simulink model "HVModAL_Fahrzeugmodell"  (R2015b)
settings: Solver=ode1  StartTime=0  StopTime=drp.driving_cycle.tstop  FixedStep=sim_params.Ts  RelTol=1e-5
PreLoadFcn:
  | % Add paths
  | addpath data
  | addpath(genpath('library'))
StartFcn:
  | Simulation.StartTime = tic;
StopFcn:
  | Simulation.DurationTime = toc(Simulation.StartTime);
undefined symbols (not defined in the file or in its folder): Batteries, BMS, BMS_Bat_, C_Nenn_DCDC1, C_Nenn_DCDC2, d2d, DC, DCDC_Converter_efficiency, DcDc_Converters, Dcl, drp, drv, elm, gen, gin, Hdc, hdc, HV, hvb, Hvb, ice, ldc, lib_dcl, lib_hdc, lib_hvb, lib_veh, Link, lossestable, mask_LUT_OCV, mask_LUT_OCV_SOC, mask_LUT_OCV_Temperature, mask_LUT_R, mask_LUT_Rs, mask_LUT_Rs_SOC, mask_LUT_Rs_Temperature, sim_params, speedvec, torquevec, tri, veh, Veh, Vehicle_Chassis
libraries: simulink x29, lib_tri_modules x7, lib_hdc_module x5, lib_gearbox x4, lib_hvb_battery_pack x3, cstblocks x3, PowerLimitBlock x2, MultiCellLibrary x2, lib_aux x1, lib_drv x1, lib_gen x1, lib_elm x1
(part 7 of 7)

== system HVModAL_Fahrzeugmodell/Energy Manager (Emg)/Battery Control/Driving_Mode/Range_extender 2/dynamic/power_distribution_new/power_follow_control ==
  note: #new#:
      | P_load-P_Bat2_max>0: --> P_load>P_Bat2_max --> P2=P_Bat2_max; P1=P_load-P2; discharge
      |
      | P_load-P_Bat2_max<0: --> 1): 0<P_load<P_Bat2_max -->P2=P_load*3; P1=P_load-P2; charged or (0<P_load<P_Bat2_max -->P2=P_load; P1=0;)
      |
      | 2): P_load<0 --> P2=|P_load|&P2<=P_Bat2_max; P1=P_load+P2; charged
  note: #previous#:
      | P_load-P_Bat2_max>0: --> P_load>P_Bat2_max --> P2=P_Bat2_max; P1=P_load-P2; discharge
      |
      | P_load-P_Bat2_max<0: --> 1): 0<P_load<P_Bat2_max -->P2=P_Bat2_max; P1=P_load-P2; charged
      |
      | 2): P_load<0 --> P2=P_Bat2_max; P1=P_load+P2; charged
  P_load : Inport
  P_Bat2_discharge_max : Inport  Port=2
  Constant1 : Constant  Value=0
  Gain : Gain  Gain=-1
  Gain1 : Gain  Gain=5
  P_Bat2_new : Scope  NumInputPorts=2
  P_Bat2_old : Scope  NumInputPorts=2
  P_UB_Bat1#2 : Scope
  Saturation1 : Saturate  UpperLimit=0  LowerLimit=-inf
  Subtract1 : Sum  Inputs=+-
  Subtract2 : Sum  Inputs=+-
  Subtract3 : Sum  Inputs=+-
  Switch{1,3..5} (4 alike) : Switch
  Switch2 : Switch  Threshold=5
  P_Bat2 : Outport
  wires:
  Switch1/1 -> P_Bat2/1, P_Bat2_new/2
  P_Bat2_discharge_max/1 -> Subtract2/2, Switch5/1, P_UB_Bat1#2/1, Switch1/1, Subtract3/2, Switch2/1
  Constant1/1 -> Switch2/3
  Switch2/1 -> Subtract1/2, Switch3/1
  Subtract1/1 -> Switch3/2
  Switch3/1 -> Switch4/1, Switch4/2
  Saturation1/1 -> Gain/1
  Gain/1 -> Switch5/3, Subtract2/1
  Subtract2/1 -> Switch5/2
  Switch5/1 -> Switch4/3
  Subtract3/1 -> Switch1/2
  Gain1/1 -> Switch1/3, Subtract3/1
  Switch4/1 -> P_Bat2_old/2, Gain1/1
  P_load/1 -> Switch2/2, Saturation1/1, Switch3/3, Subtract1/1, P_Bat2_new/1, P_Bat2_old/1

== system HVModAL_Fahrzeugmodell/Energy Manager (Emg)/Battery Control/Driving_Mode/Range_extender 2/dynamic/power_distribution_new/prevent_bat1_overcharge&& temperature control ==
  note: p_bat2_now= p_bat2 + overcharge_power (negative)
  note: Compare whether P_Bat1 beyond the limit P_max_charge
      | P_Bat1 - P_Bat1_max_charge (negative)
      | = positive --> normal charge
      | = negative --> overcharge
  note: p_bat1_max_charge (negative)
  note: P_Bat1=P_load-P_bat2
  note: <0 overcharge
  "P_load " : Inport
  P_bat2 : Inport  Port=2
  T_Cell_avg : Inport  Port=3
  Constant1 : Constant  Value=0
  Constant3 : Constant  Value=hvb.Bat1.P_max_cha
  Gain : Gain  Gain=-1
  Relational Operator4 : RelationalOperator  OutDataTypeStr=boolean
  Saturation : Saturate  UpperLimit=hvb.Bat2.P_max_disch  LowerLimit=0
  Subtract1 : Sum  Inputs=+-
  Subtract2 : Sum  Inputs=+-
  Subtract3 : Sum
  Switch1 : Switch  Criteria=u2 > Threshold
  Switch3 : Switch  Criteria=u2 > Threshold
  T_threshold : Constant  Value=-20
  "p_pat2_new " : Outport
  wires:
  Constant3/1 -> Gain/1
  Subtract2/1 -> Switch3/2, Subtract3/2
  Gain/1 -> Subtract2/2
  "P_load "/1 -> Subtract1/1
  Subtract1/1 -> Subtract2/1
  Subtract3/1 -> Saturation/1
  Saturation/1 -> Switch3/3
  P_bat2/1 -> Subtract1/2, Switch3/1, Subtract3/1
  T_threshold/1 -> Relational Operator4/2
  Relational Operator4/1 -> Switch1/2
  T_Cell_avg/1 -> Relational Operator4/1
  Switch1/1 -> "p_pat2_new "/1
  Switch3/1 -> Switch1/1
  Constant1/1 -> Switch1/3

== system HVModAL_Fahrzeugmodell/Energy Manager (Emg)/Battery Control/Driving_Mode/Range_extender 2/dynamic/soc estimination /SOC & I_rex  ==
  note: soc<30 => soc=30
  note: soc>79 => soc=100
  note: soc > 79%             convert to 100% (small difference between the effects of step-in soc 100% and 80% )
      | 79% > soc > 30%  stay
      | 30% > soc              convert to 30% (step-in soc lower than 30%, I_rex will be too high, Bat2 will be consumed too fast )
  note: To determine the current in each cell (I_rex) and the step-in soc
      | by different bat1 capacity and driving range
  E_bat1 : Inport
  speed : Inport  Port=2
  specific energy consumption : Inport  Port=3
  "cell " : Inport  Port=4
  driving range : Inport  Port=5
  Chart3 : Stateflow chart  TreatAsAtomicUnit=on
      settings: PermitHierarchicalResolution=ParametersOnly
  Constant5 : Constant  Value=100
  Constant8 : Constant  Value=30
  Display : Display
  Display1 : Display
  Saturation : Saturate  UpperLimit=hvb.Bat2.cell.I_max_disch  LowerLimit=0
  Scope{1,4,6..8,13} (6 alike) : Scope
  Switch2 : Switch  Criteria=u2 > Threshold  Threshold=79
  Switch4 : Switch  Criteria=u2 > Threshold  Threshold=30
  soc : Outport
  I_rex : Outport  Port=2
  wires:
  Constant5/1 -> Switch2/1
  Switch2/1 -> Switch4/1, Switch4/2
  Constant8/1 -> Switch4/3
  Switch4/1 -> soc/1
  speed/1 -> Chart3/2(speed)
  specific energy consumption/1 -> Chart3/3(E)
  Chart3/2(I_rex) -> Saturation/1
  Chart3/1(soc) -> Scope4/1, Switch2/3, Switch2/2
  Chart3/3(range) -> Scope6/1
  Chart3/4(range_2) -> Scope7/1
  Chart3/5(range_1) -> Scope8/1
  "cell "/1 -> Display1/1, Chart3/4(cell)
  E_bat1/1 -> Scope1/1, Chart3/1(E_bat1)
  Saturation/1 -> Scope13/1, I_rex/1
  driving range/1 -> Display/1, Chart3/5(driving_range)

== system HVModAL_Fahrzeugmodell/Energy Manager (Emg)/Battery Control/Driving_Mode/Range_extender 2/start_from_30% 1/power estimination /mapping1 ==
  P_max_ch_W_Bat1 : Inport
  P_max_Disch_W_Bat1 : Inport  Port=2
  Gain : Gain  Gain=-1
  P_LB_Bat1 : Outport
  P_UB_Bat1 : Outport  Port=2
  wires:
  Gain/1 -> P_LB_Bat1/1
  P_max_ch_W_Bat1/1 -> Gain/1
  P_max_Disch_W_Bat1/1 -> P_UB_Bat1/1

== system HVModAL_Fahrzeugmodell/Energy Manager (Emg)/Battery Control/Driving_Mode/Range_extender 2/start_from_30% 1/power_distribution_new/prevent_bat1_overcharge&& temperature control ==
  note: p_bat2_now= p_bat2_previous + overcharge_power (negative)
  note: p_bat1 - p_bat1_max_charge (negative)
      | = positive --> normal charge
      | = negative --> overcharge
  note: p_bat1_max_charge (negative)
  note: P_bat1=p_load-p_bat2
  note: <0 overcharge
  "p_load " : Inport
  p_bat2_previous : Inport  Port=2
  T_Cell_avg : Inport  Port=3
  Constant1 : Constant  Value=0
  Constant3 : Constant  Value=hvb.Bat1.P_max_cha
  Gain : Gain  Gain=-1
  Relational Operator4 : RelationalOperator  OutDataTypeStr=boolean
  Saturation : Saturate  UpperLimit=hvb.Bat2.P_max_disch  LowerLimit=0
  Scope : Scope
  Subtract1 : Sum  Inputs=+-
  Subtract2 : Sum  Inputs=+-
  Subtract3 : Sum
  Switch1 : Switch  Criteria=u2 > Threshold
  Switch3 : Switch  Criteria=u2 > Threshold
  T_threshold : Constant  Value=-20
  "p_pat2_now " : Outport
  wires:
  Constant3/1 -> Scope/1, Gain/1
  Subtract2/1 -> Switch3/2, Subtract3/2
  Gain/1 -> Subtract2/2
  "p_load "/1 -> Subtract1/1
  Subtract1/1 -> Subtract2/1
  Subtract3/1 -> Saturation/1
  Saturation/1 -> Switch3/3
  p_bat2_previous/1 -> Subtract1/2, Switch3/1, Subtract3/1
  Constant1/1 -> Switch1/3
  Relational Operator4/1 -> Switch1/2
  T_Cell_avg/1 -> Relational Operator4/1
  Switch1/1 -> "p_pat2_now "/1
  Switch3/1 -> Switch1/1
  T_threshold/1 -> Relational Operator4/2

== system HVModAL_Fahrzeugmodell/Energy Manager (Emg)/Battery Control/Driving_Mode/Range_extender 2/start_from_30% 1/soc estimination /Subsystem ==
  note: actual distance the rest capacity of bat1 can do
  note: rest distance
  soc_perc_bat1 : Inport
  E_bat1 : Inport  Port=2
  driving_range : Inport  Port=3
  V : Inport  Port=4
  % : Constant  Value=100
  5% soc rest : Constant  Value=5
  Add : Sum  Inputs=+-
  Add1 : Sum  Inputs=+-
  Constant3 : Constant  Value=1000
  Divide : Product  Inputs=*/
  Divide2 : Product  Inputs=**//
  Integrator : Integrator
  Relational Operator1 : RelationalOperator  Operator=>  OutDataTypeStr=boolean
  Scope : Scope
  energy consumption per km : Constant  Value=160
  only_bat1_capability : Outport
  wires:
  Divide/1 -> Add1/2, Scope/1
  soc_perc_bat1/1 -> Add/1
  Divide2/1 -> Relational Operator1/1
  Add1/1 -> Relational Operator1/2
  energy consumption per km/1 -> Divide2/4
  Add/1 -> Divide2/1
  %/1 -> Divide2/3
  5% soc rest/1 -> Add/2
  V/1 -> Integrator/1
  Relational Operator1/1 -> only_bat1_capability/1
  Constant3/1 -> Divide/2
  Integrator/1 -> Divide/1
  driving_range/1 -> Add1/1
  E_bat1/1 -> Divide2/2

== system HVModAL_Fahrzeugmodell/Energy Manager (Emg)/Battery Control/Driving_Mode/Range_extender 2/start_from_begining /power estimination /mapping1 ==
  P_max_ch_W_Bat1 : Inport
  P_max_Disch_W_Bat1 : Inport  Port=2
  Gain : Gain  Gain=-1
  P_LB_Bat1 : Outport
  P_UB_Bat1 : Outport  Port=2
  wires:
  Gain/1 -> P_LB_Bat1/1
  P_max_ch_W_Bat1/1 -> Gain/1
  P_max_Disch_W_Bat1/1 -> P_UB_Bat1/1

== system HVModAL_Fahrzeugmodell/Energy Manager (Emg)/Battery Control/Driving_Mode/Range_extender 2/start_from_begining /power_distribution_new/power_follow_control ==
  note: #new#:
      | P_load-P_Bat2_max>0: --> P_load>P_Bat2_max --> P2=P_Bat2_max; P1=P_load-P2; discharge
      |
      | P_load-P_Bat2_max<0: --> 1): 0<P_load<P_Bat2_max -->P2=P_load*3; P1=P_load-P2; charged or (0<P_load<P_Bat2_max -->P2=P_load; P1=0;)
      |
      | 2): P_load<0 --> P2=|P_load|&P2<=P_Bat2_max; P1=P_load+P2; charged
  note: #previous#:
      | P_load-P_Bat2_max>0: --> P_load>P_Bat2_max --> P2=P_Bat2_max; P1=P_load-P2; discharge
      |
      | P_load-P_Bat2_max<0: --> 1): 0<P_load<P_Bat2_max -->P2=P_Bat2_max; P1=P_load-P2; charged
      |
      | 2): P_load<0 --> P2=P_Bat2_max; P1=P_load+P2; charged
  P_load : Inport
  P_Bat2_discharge_max : Inport  Port=2
  Constant1 : Constant  Value=0
  Gain : Gain  Gain=-1
  Gain1 : Gain
  P_Bat2_new : Scope  NumInputPorts=2
  P_Bat2_old : Scope  NumInputPorts=2
  P_UB_Bat1#2 : Scope
  Saturation1 : Saturate  UpperLimit=0  LowerLimit=-inf
  Subtract1 : Sum  Inputs=+-
  Subtract2 : Sum  Inputs=+-
  Subtract3 : Sum  Inputs=+-
  Switch{1,3..5} (4 alike) : Switch
  Switch2 : Switch  Threshold=5
  P_Bat2 : Outport
  wires:
  Switch1/1 -> P_Bat2/1, P_Bat2_new/2
  P_Bat2_discharge_max/1 -> Subtract2/2, Switch5/1, P_UB_Bat1#2/1, Switch1/1, Subtract3/2, Switch2/1
  Constant1/1 -> Switch2/3
  Switch2/1 -> Subtract1/2, Switch3/1
  Subtract1/1 -> Switch3/2
  Switch3/1 -> Switch4/1, Switch4/2
  Saturation1/1 -> Gain/1
  Gain/1 -> Switch5/3, Subtract2/1
  Subtract2/1 -> Switch5/2
  Switch5/1 -> Switch4/3
  Subtract3/1 -> Switch1/2
  Gain1/1 -> Switch1/3, Subtract3/1
  Switch4/1 -> P_Bat2_old/2, Gain1/1
  P_load/1 -> Switch2/2, Saturation1/1, Switch3/3, Subtract1/1, P_Bat2_new/1, P_Bat2_old/1

== system HVModAL_Fahrzeugmodell/Energy Manager (Emg)/Battery Control/Driving_Mode/Range_extender 2/start_from_begining /power_distribution_new/prevent_bat1_overcharge&& temperature control ==
  note: p_bat2_new= p_bat2_old + overcharge_power (negative)
  note: p_bat1 - p_bat1_max_charge (negative)
      | = positive --> normal charge
      | = negative --> overcharge
  note: p_bat1_max_charge (negative)
  note: P_bat1=p_load-p_bat2
  note: <0 overcharge
  "p_load " : Inport
  p_bat2_old : Inport  Port=2
  T_Cell_avg : Inport  Port=3
  Constant1 : Constant  Value=0
  Constant3 : Constant  Value=hvb.Bat1.P_max_cha
  Gain : Gain  Gain=-1
  Relational Operator4 : RelationalOperator  OutDataTypeStr=boolean
  Saturation : Saturate  UpperLimit=hvb.Bat2.P_max_disch  LowerLimit=0
  Subtract1 : Sum  Inputs=+-
  Subtract2 : Sum  Inputs=+-
  Subtract3 : Sum
  Switch1 : Switch  Criteria=u2 > Threshold
  Switch3 : Switch  Criteria=u2 > Threshold
  T_threshold : Constant  Value=-20
  "p_pat2_new " : Outport
  wires:
  Constant3/1 -> Gain/1
  Subtract2/1 -> Switch3/2, Subtract3/2
  Gain/1 -> Subtract2/2
  "p_load "/1 -> Subtract1/1
  Subtract1/1 -> Subtract2/1
  Subtract3/1 -> Saturation/1
  Saturation/1 -> Switch3/3
  p_bat2_old/1 -> Subtract1/2, Switch3/1, Subtract3/1
  Constant1/1 -> Relational Operator4/2
  Relational Operator4/1 -> Switch1/2
  T_Cell_avg/1 -> Relational Operator4/1
  Switch1/1 -> "p_pat2_new "/1
  Switch3/1 -> Switch1/1
  T_threshold/1 -> Switch1/3

== system HVModAL_Fahrzeugmodell/Energy Manager (Emg)/Battery Control/Driving_Mode/Strategy_Maximiziation_Driving_Range1/Minloss Strategy/Sufficient Energy left/SOC Management ==
  Pload : Inport
  R1 : Inport  Port=2
  R2 : Inport  Port=3
  V1 : Inport  Port=4
  V2 : Inport  Port=5
  P_max_disch_bat1 : Inport  Port=6
  P_max_char_bat2 : Inport  Port=7
  P_max_disch_bat2 : Inport  Port=8
  P_max_char_bat1 : Inport  Port=9
  Enable : EnablePort
  Acceleration : Subsystem
  Compare To Zero : simulink/Logic and Bit Operations/Compare To Zero  relop=>  OutDataTypeStr=boolean
  L : Logic  Operator=NOT  AllPortsSameDT=off  OutDataTypeStr=boolean
  Merge : Merge
  Merge1 : Merge
  Recuperation : Subsystem
  vector_PowerDistribution : Outport
  P_exchange_Master_Slave : Outport  Port=2
  wires:
  Recuperation/2(P_exchange_Master_Slave) -> Merge1/2
  Acceleration/2(P_exchange_Master_Slave) -> Merge1/1
  Merge1/1 -> P_exchange_Master_Slave/1
  Merge/1 -> vector_PowerDistribution/1
  Pload/1 -> Compare To Zero/1, Recuperation/5(Pload)
  P_max_char_bat2/1 -> Acceleration/6(P_max_char_bat2), Recuperation/2(P_max_char_bat2)
  P_max_char_bat1/1 -> Recuperation/4(P_max_char_bat1)
  P_max_disch_bat2/1 -> Recuperation/3(P_max_disch_bat2)
  Recuperation/1(vector_PowerDistribution) -> Merge/2
  L/1 -> Recuperation/Enable
  Compare To Zero/1 -> Acceleration/Enable, L/1
  Acceleration/1(vector_PowerDistribution) -> Merge/1
  P_max_disch_bat1/1 -> Acceleration/5(P_max_disch_bat1), Recuperation/1(P_max_disch_bat1)
  V2/1 -> Acceleration/4(V2)
  V1/1 -> Acceleration/3(V1)
  R2/1 -> Acceleration/2(R2)
  R1/1 -> Acceleration/1(R1)

== system HVModAL_Fahrzeugmodell/Energy Manager (Emg)/Battery Control/Driving_Mode/Strategy_Maximiziation_Driving_Range1/Minloss Strategy/Sufficient Energy left/SOC Management/Acceleration ==
  R1 : Inport
  R2 : Inport  Port=2
  V1 : Inport  Port=3
  V2 : Inport  Port=4
  P_max_disch_bat1 : Inport  Port=5
  P_max_char_bat2 : Inport  Port=6
  Enable : EnablePort
  Constant : Constant  Value=0
  Constant1 : Constant
  Constant2 : Constant  Value=0
  Gain : Gain  Gain=100
  Mux1 : Mux  Inputs=3
  N : Constant  Value=50
  Optimal charge power : Subsystem  TreatAsAtomicUnit=on
  vector_PowerDistribution : Outport
  P_exchange_Master_Slave : Outport  Port=2
  wires:
  Gain/1 -> vector_PowerDistribution/1
  Constant1/1 -> Mux1/1
  N/1 -> Optimal charge power/7(N)
  V2/1 -> Optimal charge power/4(V2)
  P_max_disch_bat1/1 -> Optimal charge power/5(P_max_disch_bat1)
  Mux1/1 -> Gain/1
  Constant2/1 -> Mux1/2
  R1/1 -> Optimal charge power/1("R1 ")
  Optimal charge power/1(P_trans) -> P_exchange_Master_Slave/1  "P_transferred"
  R2/1 -> Optimal charge power/2("R2 ")
  Constant/1 -> Mux1/3  "powershare_bat3"
  P_max_char_bat2/1 -> Optimal charge power/6(P_max_char_bat2)
  V1/1 -> Optimal charge power/3(V1)

== system HVModAL_Fahrzeugmodell/Energy Manager (Emg)/Battery Control/Driving_Mode/Strategy_Maximiziation_Driving_Range1/Minloss Strategy/Sufficient Energy left/SOC Management/Recuperation ==
  P_max_disch_bat1 : Inport
  P_max_char_bat2 : Inport  Port=2
  P_max_disch_bat2 : Inport  Port=3
  P_max_char_bat1 : Inport  Port=4
  Pload : Inport  Port=5
  Enable : EnablePort
  Constant : Constant  Value=0
  Constant1 : Constant  Value=0
  Constant2 : Constant
  Constant3 : Constant  Value=0
  Gain : Gain  Gain=100
  Mux1 : Mux  Inputs=3
  Power Limit1 : PowerLimitBlock/Power Limit
  Saturation : Saturate  UpperLimit=-0.001  LowerLimit=-inf
  vector_PowerDistribution : Outport
  P_exchange_Master_Slave : Outport  Port=2
  wires:
  Constant3/1 -> P_exchange_Master_Slave/1
  Gain/1 -> vector_PowerDistribution/1
  Saturation/1 -> Power Limit1/7
  Constant2/1 -> Power Limit1/6
  Constant1/1 -> Power Limit1/5
  Pload/1 -> Saturation/1
  Constant/1 -> Mux1/3
  Power Limit1/2 -> Mux1/2
  Power Limit1/1 -> Mux1/1
  P_max_char_bat1/1 -> Power Limit1/2
  P_max_disch_bat2/1 -> Power Limit1/3
  P_max_char_bat2/1 -> Power Limit1/4
  P_max_disch_bat1/1 -> Power Limit1/1
  Mux1/1 -> Gain/1

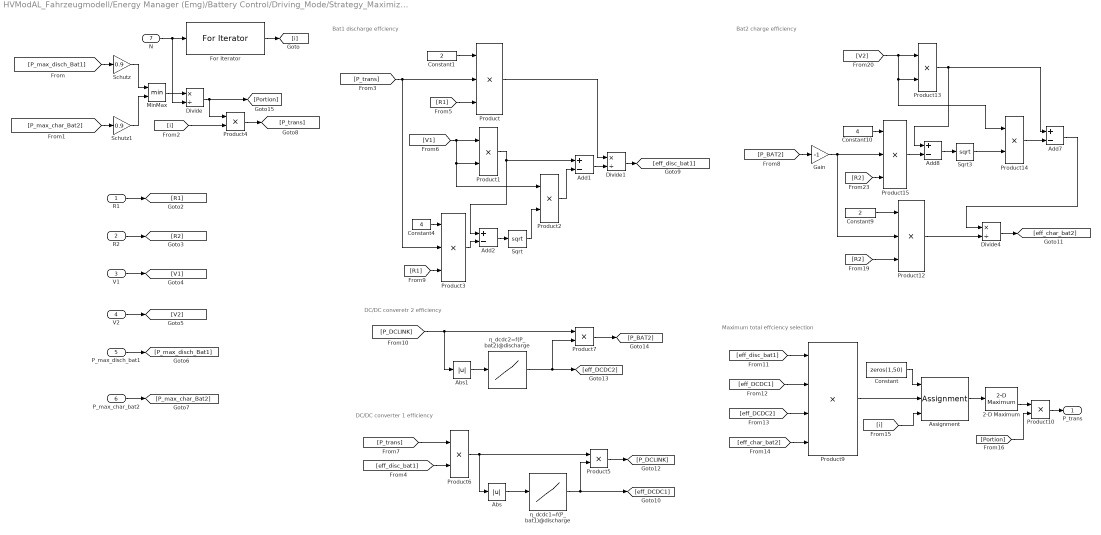
== system HVModAL_Fahrzeugmodell/Energy Manager (Emg)/Battery Control/Driving_Mode/Strategy_Maximiziation_Driving_Range1/Minloss Strategy/Sufficient Energy left/SOC Management/Acceleration/Optimal charge power ==
  note: Bat1 discharge effciency
  note: Bat2 charge efficiency
  note: Maximum total effciency selection
  note: DC/DC converter 1 efficiency
  note: DC/DC converetr 2 efficiency
  "R1 " : Inport
  "R2 " : Inport  Port=2
  V1 : Inport  Port=3
  V2 : Inport  Port=4
  P_max_disch_bat1 : Inport  Port=5
  P_max_char_bat2 : Inport  Port=6
  N : Inport  Port=7
  2-D Maximum : visionstatistics/2-D Maximum  fcn=Value and Index  reset=None  indexBase=One  operateOver=Entire input  Dimension=1  colComp=on  operation=maximum  roiEnable=off  roiType=Rectangles  roiPortion=Entire ROI  roiOutput=Individual statistics for each ROI  roiFlag=off  accumDataTypeStr=Inherit: Same as product output  accumLastDataTypeStr=Inherit: Same as product output  roundingMode=Floor  overflowMode=off
  Abs : Abs
  Abs1 : Abs
  Add{1..2,7..8} (4 alike) : Sum  Inputs=+-
  Assignment : Assignment  DiagnosticForDimensions=Warning  IndexOptions=Index vector (port)  Indices=1  OutputSizes=1
  Constant : Constant  Value=zeros(1,50)
  Constant1 : Constant  Value=2
  Constant10 : Constant  Value=4
  Constant4 : Constant  Value=4
  Constant9 : Constant  Value=2
  Divide : Product  Inputs=*/
  Divide1 : Product  Inputs=*/
  Divide4 : Product  Inputs=*/
  For Iterator : ForIterator  IterationSource=external
  Gain : Gain  Gain=-1
  MinMax : MinMax  Inputs=2
  Product{,3,12,15} (4 alike) : Product  Inputs=3
  Product{1..2,4..7,10,13..14} (9 alike) : Product
  Product9 : Product  Inputs=4
  Schutz : Gain  Gain=0.9
  Schutz1 : Gain  Gain=0.9
  Sqrt : Sqrt  SaturateOnIntegerOverflow=on
  Sqrt3 : Sqrt  SaturateOnIntegerOverflow=on
  η_dcdc1=f(P_bat1)@discharge : Lookup_n-D  NumberOfTableDimensions=1  BreakpointsForDimension1=DCDC_Converter_efficiency(1,1:8)*C_Nenn_DCDC1  Table=DCDC_Converter_efficiency(2,1:8)  ExtrapMethod=Clip  UseLastTableValue=on  InternalRulePriority=Speed  RndMeth=Simplest  InputSameDT=on
  η_dcdc2=f(P_bat2)@discharge : Lookup_n-D  NumberOfTableDimensions=1  BreakpointsForDimension1=DCDC_Converter_efficiency(1,1:8)*C_Nenn_DCDC2  Table=DCDC_Converter_efficiency(2,1:8)  ExtrapMethod=Clip  UseLastTableValue=on  InternalRulePriority=Speed  RndMeth=Simplest  InputSameDT=on
  P_trans : Outport
  wires:
  Add1/1 -> Divide1/2
  Add2/1 -> Sqrt/1
  Divide4/1 -> [eff_char_bat2]
  Gain/1 -> Product15/2, Product12/2
  Product6/1 -> Product5/1, Abs/1
  Abs/1 -> η_dcdc1=f(P_bat1)@discharge/1
  Product4/1 -> [P_trans]
  [eff_char_bat2] -> Product9/4
  [eff_DCDC2] -> Product9/3
  [eff_DCDC1] -> Product9/2
  Product10/1 -> P_trans/1
  [Portion] -> Product10/2
  2-D Maximum/2 -> Product10/1
  Assignment/1 -> 2-D Maximum/1
  Constant/1 -> Assignment/1
  [i] -> Assignment/3
  Product9/1 -> Assignment/2
  [eff_disc_bat1] -> Product9/1
  Product7/1 -> [P_BAT2]
  [P_DCLINK] -> Product7/1, Abs1/1
  η_dcdc2=f(P_bat2)@discharge/1 -> Product7/2, [eff_DCDC2]
  Abs1/1 -> η_dcdc2=f(P_bat2)@discharge/1
  [P_trans] -> Product6/1
  [eff_disc_bat1] -> Product6/2
  Product5/1 -> [P_DCLINK]
  η_dcdc1=f(P_bat1)@discharge/1 -> Product5/2, [eff_DCDC1]
  [i] -> Product4/2
  Divide/1 -> Product4/1, [Portion]
  MinMax/1 -> Divide/1
  Schutz1/1 -> MinMax/2
  Schutz/1 -> MinMax/1
  [P_max_char_Bat2] -> Schutz1/1
  [P_max_disch_Bat1] -> Schutz/1
  P_max_char_bat2/1 -> [P_max_char_Bat2]
  P_max_disch_bat1/1 -> [P_max_disch_Bat1]
  Divide1/1 -> [eff_disc_bat1]
  Constant1/1 -> Product/1
  Product12/1 -> Divide4/2
  Add7/1 -> Divide4/1
  [R2] -> Product15/3
  Constant10/1 -> Product15/1
  Product15/1 -> Add8/2
  Add8/1 -> Sqrt3/1
  Sqrt3/1 -> Product14/2
  Product14/1 -> Add7/2
  Product13/1 -> Add7/1, Add8/1
  [V2] -> Product13/2, Product14/1, Product13/1
  [R2] -> Product12/3
  [P_BAT2] -> Gain/1
  Constant9/1 -> Product12/1
  [R1] -> Product3/3
  Constant4/1 -> Product3/1
  [P_trans] -> Product/2, Product3/2
  Product3/1 -> Add2/2
  Sqrt/1 -> Product2/2
  Product2/1 -> Add1/2
  Product1/1 -> Add2/1, Add1/1
  [V1] -> Product1/1, Product1/2, Product2/1
  [R1] -> Product/3
  Product/1 -> Divide1/1
  V2/1 -> [V2]
  V1/1 -> [V1]
  "R2 "/1 -> [R2]
  "R1 "/1 -> [R1]
  For Iterator/1 -> [i]
  N/1 -> Divide/2, For Iterator/1

== stateflow chart HVModAL_Fahrzeugmodell/Energy Manager (Emg)/Battery Control/Driving_Mode/Range_extender 1/Chart ==
  state start
    during:Use_Range_extender=0;
  state Not_use_Range_Extender
    during: Use_Range_extender=0;
  state Check_SOC_of_Battery_01
  state Check_SOC_of_Battery_02
  state Use_Range_Extender
    during: Use_Range_extender=1;
  (default) -> start
  start -> Check_SOC_of_Battery_01
  Check_SOC_of_Battery_01 -> Not_use_Range_Extender [order 2] : [SOC_perc_01>SOC_limit]
      | {Use_Range_extender=0;}
  Not_use_Range_Extender -> Check_SOC_of_Battery_02 : [SOC_perc_01<=SOC_limit]
  Use_Range_Extender -> Not_use_Range_Extender : [SOC_perc_01>(SOC_limit+1)]
      | {Use_Range_extender=0;}
  Check_SOC_of_Battery_02 -> Not_use_Range_Extender [order 2] : [SOC_perc_02==0]
      | {Use_Range_extender=0;}
  Check_SOC_of_Battery_01 -> Check_SOC_of_Battery_02 [order 1] : [SOC_perc_01<=SOC_limit]
  Check_SOC_of_Battery_02 -> Use_Range_Extender [order 1] : [SOC_perc_02>0]
      | {Use_Range_extender=1;}
  data: SOC_perc_01 input; Use_Range_extender output; SOC_perc_02 input; SOC_limit input
  events: event local FUNCTION_CALL_EVENT

== stateflow chart HVModAL_Fahrzeugmodell/Energy Manager (Emg)/Battery Control/Driving_Mode/Range_extender 1/power_distribution_old/Chart ==
  state start
    during:P_Bat1=p_Bat1_o;
  state P_LB_Bat1
  state P_UB_Bat1
  (default) -> start
  P_UB_Bat1 -> start [order 1] : [p_Bat1_o<P_UB_Bat1&&...
      | p_Bat1_o>P_LB_Bat1]
      | {P_Bat1=p_Bat1_o;}
  start -> P_UB_Bat1 [order 1] : [p_Bat1_o>P_UB_Bat1]
      | {P_Bat1=P_UB_Bat1;}
  start -> P_LB_Bat1 [order 2] : [p_Bat1_o<P_LB_Bat1]
      | {P_Bat1=P_LB_Bat1;}
  P_LB_Bat1 -> start [order 1] : [p_Bat1_o>P_LB_Bat1&&...
      | p_Bat1_o<P_UB_Bat1]
      | {P_Bat1=p_Bat1_o;}
  P_LB_Bat1 -> P_UB_Bat1 [order 2] : [p_Bat1_o>P_UB_Bat1]
      | {P_Bat1=P_UB_Bat1;}
  P_UB_Bat1 -> P_LB_Bat1 [order 2] : [p_Bat1_o<P_LB_Bat1]
      | {P_Bat1=P_LB_Bat1;}
  data: p_Bat1_o input; P_Bat1 output; P_UB_Bat1 input; P_LB_Bat1 input
  events: event local FUNCTION_CALL_EVENT

== stateflow chart HVModAL_Fahrzeugmodell/Energy Manager (Emg)/Battery Control/Driving_Mode/Range_extender 2/start_from_begining /power_distribution_new/Chart ==
  state start
    during:P_Bat1=p_Bat1_o;
  state P_LB_Bat1
  state P_UB_Bat1
  (default) -> start
  P_UB_Bat1 -> start [order 1] : [p_Bat1_o<P_UB_Bat1&&...
      | p_Bat1_o>P_LB_Bat1]
      | {P_Bat1=p_Bat1_o;}
  start -> P_UB_Bat1 [order 1] : [p_Bat1_o>P_UB_Bat1]
      | {P_Bat1=P_UB_Bat1;}
  start -> P_LB_Bat1 [order 2] : [p_Bat1_o<P_LB_Bat1]
      | {P_Bat1=P_LB_Bat1;}
  P_LB_Bat1 -> start [order 1] : [p_Bat1_o>P_LB_Bat1&&...
      | p_Bat1_o<P_UB_Bat1]
      | {P_Bat1=p_Bat1_o;}
  P_LB_Bat1 -> P_UB_Bat1 [order 2] : [p_Bat1_o>P_UB_Bat1]
      | {P_Bat1=P_UB_Bat1;}
  P_UB_Bat1 -> P_LB_Bat1 [order 2] : [p_Bat1_o<P_LB_Bat1]
      | {P_Bat1=P_LB_Bat1;}
  data: p_Bat1_o input; P_Bat1 output; P_UB_Bat1 input; P_LB_Bat1 input
  events: event local FUNCTION_CALL_EVENT

== stateflow chart HVModAL_Fahrzeugmodell/Energy Manager (Emg)/Battery Control/Driving_Mode/Range_extender 2/start_from_30% 1/power_distribution_new/Chart ==
  state start
    during:P_Bat1=p_Bat1_o;
  state P_LB_Bat1
  state P_UB_Bat1
  (default) -> start
  P_UB_Bat1 -> start [order 1] : [p_Bat1_o<P_UB_Bat1&&...
      | p_Bat1_o>P_LB_Bat1]
      | {P_Bat1=p_Bat1_o;}
  start -> P_UB_Bat1 [order 1] : [p_Bat1_o>P_UB_Bat1]
      | {P_Bat1=P_UB_Bat1;}
  start -> P_LB_Bat1 [order 2] : [p_Bat1_o<P_LB_Bat1]
      | {P_Bat1=P_LB_Bat1;}
  P_LB_Bat1 -> start [order 1] : [p_Bat1_o>P_LB_Bat1&&...
      | p_Bat1_o<P_UB_Bat1]
      | {P_Bat1=p_Bat1_o;}
  P_LB_Bat1 -> P_UB_Bat1 [order 2] : [p_Bat1_o>P_UB_Bat1]
      | {P_Bat1=P_UB_Bat1;}
  P_UB_Bat1 -> P_LB_Bat1 [order 2] : [p_Bat1_o<P_LB_Bat1]
      | {P_Bat1=P_LB_Bat1;}
  data: p_Bat1_o input; P_Bat1 output; P_UB_Bat1 input; P_LB_Bat1 input
  events: event local FUNCTION_CALL_EVENT

== stateflow chart HVModAL_Fahrzeugmodell/Energy Manager (Emg)/Battery Control/Driving_Mode/Range_extender 2/dynamic/soc estimination /Chart3 ==
  (default) -> (junction 52) : % while
  (junction 52) -> (junction 54) : {i=10;...
      | range=0;}
  (junction 54) -> (junction 53) [order 1] : [range<driving_range&&i<101]
  (junction 53) -> (junction 55) : {soc=i;...
      |  rest=soc*E_bat1/100;...
      |  range_1=rest/E;...
      | range_bat1=E_bat1/E;...
      |  t=range_1/speed;...
      |  I_rex=3.1/t;...
      |  e_rex=1/(0.216+0.0479*I_rex)*cell;...
      |  range_2=e_rex/E;...
      |  range=range_bat1+range_2;...
      |  i=i+10;  }
  (junction 55) -> (junction 54)
  (junction 54) -> (junction 56) [order 2]
  data: E_bat1 input; speed input; E input; cell input; t local; e_rex local; E_rex local; rest local; soc output; I_rex output; range output; i local; range_2 output; range_1 output; range_bat1 local; driving_range input

== stateflow chart HVModAL_Fahrzeugmodell/Energy Manager (Emg)/Battery Control/Driving_Mode/Range_extender 2/dynamic/power_distribution_new/Chart ==
  state start
    during:P_Bat1=p_Bat1_o;
  state P_LB_Bat1
  state P_UB_Bat1
  (default) -> start
  P_UB_Bat1 -> start [order 1] : [p_Bat1_o<P_UB_Bat1&&...
      | p_Bat1_o>P_LB_Bat1]
      | {P_Bat1=p_Bat1_o;}
  start -> P_UB_Bat1 [order 1] : [p_Bat1_o>P_UB_Bat1]
      | {P_Bat1=P_UB_Bat1;}
  start -> P_LB_Bat1 [order 2] : [p_Bat1_o<P_LB_Bat1]
      | {P_Bat1=P_LB_Bat1;}
  P_LB_Bat1 -> start [order 1] : [p_Bat1_o>P_LB_Bat1&&...
      | p_Bat1_o<P_UB_Bat1]
      | {P_Bat1=p_Bat1_o;}
  P_LB_Bat1 -> P_UB_Bat1 [order 2] : [p_Bat1_o>P_UB_Bat1]
      | {P_Bat1=P_UB_Bat1;}
  P_UB_Bat1 -> P_LB_Bat1 [order 2] : [p_Bat1_o<P_LB_Bat1]
      | {P_Bat1=P_LB_Bat1;}
  data: p_Bat1_o input; P_Bat1 output; P_UB_Bat1 input; P_LB_Bat1 input
  events: event local FUNCTION_CALL_EVENT

== stateflow chart HVModAL_Fahrzeugmodell/Energy Manager (Emg)/Battery Control/Driving_Mode/Range_extender 1/power_distribution_new/Chart ==
  state start
    during:P_Bat1=p_Bat1_o;
  state P_LB_Bat1
  state P_UB_Bat1
  (default) -> start
  P_UB_Bat1 -> start [order 1] : [p_Bat1_o<P_UB_Bat1&&...
      | p_Bat1_o>P_LB_Bat1]
      | {P_Bat1=p_Bat1_o;}
  start -> P_UB_Bat1 [order 1] : [p_Bat1_o>P_UB_Bat1]
      | {P_Bat1=P_UB_Bat1;}
  start -> P_LB_Bat1 [order 2] : [p_Bat1_o<P_LB_Bat1]
      | {P_Bat1=P_LB_Bat1;}
  P_LB_Bat1 -> start [order 1] : [p_Bat1_o>P_LB_Bat1&&...
      | p_Bat1_o<P_UB_Bat1]
      | {P_Bat1=p_Bat1_o;}
  P_LB_Bat1 -> P_UB_Bat1 [order 2] : [p_Bat1_o>P_UB_Bat1]
      | {P_Bat1=P_UB_Bat1;}
  P_UB_Bat1 -> P_LB_Bat1 [order 2] : [p_Bat1_o<P_LB_Bat1]
      | {P_Bat1=P_LB_Bat1;}
  data: p_Bat1_o input; P_Bat1 output; P_UB_Bat1 input; P_LB_Bat1 input
  events: event local FUNCTION_CALL_EVENT

== stateflow chart HVModAL_Fahrzeugmodell/Energy Manager (Emg)/Battery Control/Driving_Mode/Range_extender 2/dynamic/soc estimination /Chart ==
  state start
    during:Use_Range_extender=0;
  state Check_SOC_of_Battery_01
  state Not_use_Range_Extender
    during: Use_Range_extender=0;
  state Check_SOC_of_Battery_02
  state Use_Range_Extender
    during: Use_Range_extender=1;
  (default) -> start [order 1]
  start -> Check_SOC_of_Battery_01
  (default) -> Not_use_Range_Extender [order 2] : [SOC_perc_01>SOC_limit]
      | {Use_Range_extender=0;}
  Check_SOC_of_Battery_01 -> Check_SOC_of_Battery_02 : [SOC_perc_01<=SOC_limit]
  Not_use_Range_Extender -> Check_SOC_of_Battery_02 : [SOC_perc_01<=SOC_limit]
  Check_SOC_of_Battery_02 -> Not_use_Range_Extender [order 2] : [SOC_perc_02==0]
      | {Use_Range_extender=0;}
  Check_SOC_of_Battery_02 -> Use_Range_Extender [order 1] : [SOC_perc_02>0]
      | {Use_Range_extender=1;}
  Use_Range_Extender -> Not_use_Range_Extender : [SOC_perc_01>(SOC_limit+1)]
      | {Use_Range_extender=0;}
  data: SOC_perc_01 input; Use_Range_extender output; SOC_perc_02 input; SOC_limit input
  events: event local FUNCTION_CALL_EVENT

== stateflow chart HVModAL_Fahrzeugmodell/Energy Manager (Emg)/Battery Control/Driving_Mode/Range_extender 2/dynamic/soc estimination /SOC & I_rex /Chart3 ==
  (default) -> (junction 52) : % while
  (junction 52) -> (junction 54) : {i=10;...
      | range=0;}
  (junction 54) -> (junction 53) [order 1] : [range<driving_range&&i<101]
  (junction 53) -> (junction 55) : {soc=i;...
      |  rest=soc*E_bat1/100;...
      |  range_1=rest/E;...
      | range_bat1=E_bat1/E;...
      |  t=range_1/speed;...
      |  I_rex=3.1/t;...
      |  e_rex=1/(0.216+0.0479*I_rex)*cell;...
      |  range_2=e_rex/E;...
      |  range=range_bat1+range_2;...
      |  i=i+10;  }
  (junction 55) -> (junction 54)
  (junction 54) -> (junction 56) [order 2]
  data: E_bat1 input; speed input; E input; cell input; t local; e_rex local; E_rex local; rest local; soc output; I_rex output; range output; i local; range_2 output; range_1 output; range_bat1 local; driving_range input

== stateflow chart HVModAL_Fahrzeugmodell/Energy Manager (Emg)/Battery Control/Driving_Mode/Range_extender 1/power_distribution_new/Chart2 ==
  state start
    during:p_bat2_w=p_bat2_discharge_w;
  state p_load_w
  (default) -> start
  p_load_w -> start : [p_bat2_discharge_w<p_load_w|...
      | p_load_w<5]
      | {p_bat2_w=p_bat2_discharge_w;}
  start -> p_load_w : [p_bat2_discharge_w>p_load_w&&...
      | p_load_w>5 ]
      | {p_bat2_w=p_load_w;}
  data: p_load_w input; p_bat2_w output; p_bat2_discharge_w input
  events: event local FUNCTION_CALL_EVENT

== stateflow chart HVModAL_Fahrzeugmodell/Energy Manager (Emg)/Battery Control/Driving_Mode/Range_extender 1/Chart3 ==
  (default) -> (junction 52) : % while
  (junction 52) -> (junction 54) : {i=10;...
      | range=0;}
  (junction 54) -> (junction 53) [order 1] : [range<250&&i<101]
  (junction 53) -> (junction 55) : {soc=i;...
      |  rest=soc*E_bat1/100;...
      |  range_1=rest/E;...
      | range_bat1=E_bat1/E;...
      |  t=range_1/speed;...
      |  I_rex=3.1/t;...
      |  e_rex=1/(0.216+0.0479*I_rex)*cell;...
      |  range_2=e_rex/E;...
      |  range=range_bat1+range_2;...
      |  i=i+10;  }
  (junction 55) -> (junction 54)
  (junction 54) -> (junction 56) [order 2]
  data: E_bat1 input; speed input; E input; cell input; t local; e_rex local; E_rex local; rest local; soc output; I_rex output; range output; i local; range_2 output; range_1 output; range_bat1 local

== stateflow chart HVModAL_Fahrzeugmodell/Energy Manager (Emg)/Battery Control/Driving_Mode/Range_extender 1/Chart1 ==
  (default) -> (junction 52) : % while
  (junction 52) -> (junction 54) : {i=10;...
      | range=0;}
  (junction 54) -> (junction 53) [order 1] : [range<250&&i<101]
  (junction 53) -> (junction 55) : {soc=i;...
      |  rest=soc*E_bat1/100;...
      |  range_1=rest/E;...
      | range_bat1=E_bat1/E;...
      |  t=range_1/speed;...
      |  I_rex=3.1/t;...
      |  e_rex=1/(0.216+0.0479*I_rex)*cell;...
      |  range_2=e_rex/E;...
      |  range=range_bat1+range_2;...
      |  i=i+10;  }
  (junction 55) -> (junction 54)
  (junction 54) -> (junction 56) [order 2]
  data: E_bat1 input; speed input; E input; cell input; t local; e_rex local; E_rex local; rest local; soc output; I_rex output; range output; i local; range_2 output; range_1 output; range_bat1 local

== stateflow chart HVModAL_Fahrzeugmodell/Energy Manager (Emg)/Battery Control/Driving_Mode/Range_extender 2/start_from_30% 1/soc estimination /Chart ==
  state start
    during:Use_Range_extender=0;
  state Not_use_Range_Extender
    during: Use_Range_extender=0;
  state Check_SOC_of_Battery_01
  state Check_SOC_of_Battery_02
  state Use_Range_Extender
    during: Use_Range_extender=1;
  (default) -> start
  start -> Check_SOC_of_Battery_01
  Check_SOC_of_Battery_01 -> Not_use_Range_Extender [order 2] : [SOC_perc_01>SOC_limit]
      | {Use_Range_extender=0;}
  Not_use_Range_Extender -> Check_SOC_of_Battery_02 : [SOC_perc_01<=SOC_limit&&...
      | only_bat1_capability ==0]
  Use_Range_Extender -> Not_use_Range_Extender : [SOC_perc_01>(SOC_limit+1) ||...
      |  only_bat1_capability ==1]
      | {Use_Range_extender=0;}
  Check_SOC_of_Battery_02 -> Not_use_Range_Extender [order 2] : [SOC_perc_02==0]
      | {Use_Range_extender=0;}
  Check_SOC_of_Battery_01 -> Check_SOC_of_Battery_02 [order 1] : [SOC_perc_01<=SOC_limit &&...
      | only_bat1_capability ==0]
  Check_SOC_of_Battery_02 -> Use_Range_Extender [order 1] : [SOC_perc_02>0]
      | {Use_Range_extender=1;}
  data: SOC_perc_01 input; Use_Range_extender output; SOC_perc_02 input; SOC_limit input; only_bat1_capability input
  events: event local FUNCTION_CALL_EVENT

== stateflow chart HVModAL_Fahrzeugmodell/Energy Manager (Emg)/Battery Control/Driving_Mode/Range_extender 2/start_from_begining /soc estimination /Chart ==
  state start
    during:Use_Range_extender=0;
  state Check_SOC_of_Battery_01
  state Not_use_Range_Extender
    during: Use_Range_extender=0;
  state Check_SOC_of_Battery_02
  state Use_Range_Extender
    during: Use_Range_extender=1;
  (default) -> start
  start -> Check_SOC_of_Battery_01
  Check_SOC_of_Battery_01 -> Not_use_Range_Extender [order 2] : [SOC_perc_01>SOC_limit]
      | {Use_Range_extender=0;}
  Check_SOC_of_Battery_01 -> Check_SOC_of_Battery_02 [order 1] : [SOC_perc_01<=SOC_limit]
  Not_use_Range_Extender -> Check_SOC_of_Battery_02 : [SOC_perc_01<=SOC_limit]
  Check_SOC_of_Battery_02 -> Not_use_Range_Extender [order 2] : [SOC_perc_02==0]
      | {Use_Range_extender=0;}
  Check_SOC_of_Battery_02 -> Use_Range_Extender [order 1] : [SOC_perc_02>0]
      | {Use_Range_extender=1;}
  Use_Range_Extender -> Not_use_Range_Extender : [SOC_perc_01>(SOC_limit+1)]
      | {Use_Range_extender=0;}
  data: SOC_perc_01 input; Use_Range_extender output; SOC_perc_02 input; SOC_limit input
  events: event local FUNCTION_CALL_EVENT
